simulink model "PID_Controller"  (R2020b)
settings: Solver=VariableStepAuto  StartTime=0.0  StopTime=10.0  RelTol=1e-3
model workspace (MAT data in the model file):
  J = 3.2284e-06
  K = 0.0274
  L = 2.75e-06
  R = 4
  b = 3.5077e-06
settings Model: Creator=sai  LastModifiedBy=sai
settings DataIOCC: SaveOutput=off  SaveTime=off

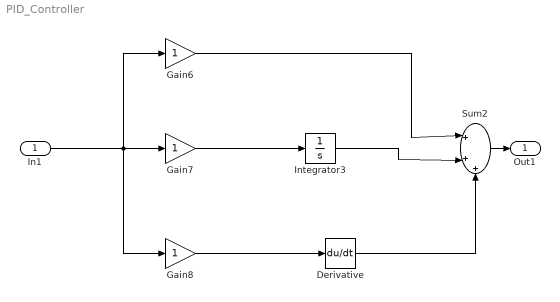
== system PID_Controller ==
  In1 : Inport  OutDataTypeStr=double  PortDimensions=1  SampleTime=0
  Derivative : Derivative
  Gain6 : Gain
  Gain7 : Gain
  Gain8 : Gain
  Integrator3 : Integrator
  Sum2 : Sum  Inputs=|+++
  Out1 : Outport  OutDataTypeStr=double  PortDimensions=1  SampleTime=0
  wires:
  Gain8/1 -> Derivative/1
  In1/1 -> Gain7/1, Gain6/1, Gain8/1
  Sum2/1 -> Out1/1
  Derivative/1 -> Sum2/3
  Integrator3/1 -> Sum2/2
  Gain6/1 -> Sum2/1
  Gain7/1 -> Integrator3/1
